simulink model "sldemo_foucault"  (Simulink 10.0)
settings: Solver=ode23t  StartTime=0.0  StopTime=3600  FixedStep=.1  RelTol=1e-5  EnableMultiTasking=on
PreLoadFcn:
  | sldemo_foucault_data;
undefined symbols (not defined in the file): g, initial_x, initial_xdot, initial_y, initial_ydot, L, lambda, Omega
CloseFcn:
  | close(findobj('Tag','CloseMe'));
settings Model: Creator=The MathWorks, Inc.  LastModifiedBy=bhisma
settings DataIOCC: SaveFormat=StructureWithTime  SaveOutput=off  SaveTime=off  ReturnWorkspaceOutputs=on  ReturnWorkspaceOutputsName=sldemo_foucault_output
settings OptimizationCC: ExpressionDepthLimit=2147483647  InitFltsAndDblsToZero=on
settings DebuggingCC: SaveWithParameterizedLinksMsg=none  SignalResolutionControl=TryResolveAllWithWarning  FcnCallInpInsideContextMsg=warning  AllowSymbolicDim=off  StateNameClashWarn=warning
settings SFSimCC: CustomCodeUndefinedFunction=FilterOut
settings GRTTargetCC: TargetFcnLib=ansi_tfl_tmw.mat  GeneratePreprocessorConditionals=Disable all
settings ConfigComp: CovExternalEMLEnable=off

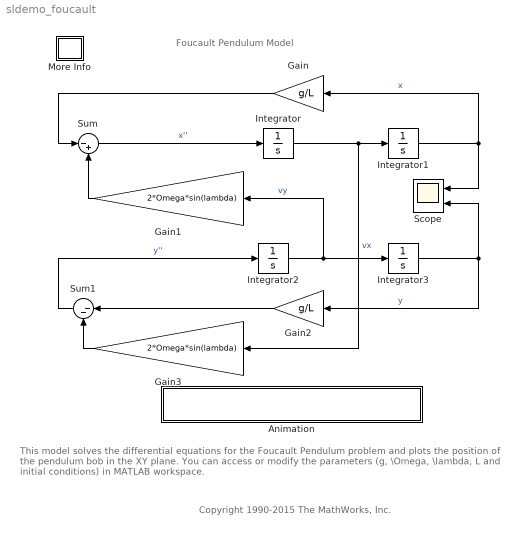
== system sldemo_foucault ==
  note: This model solves the differential equations for the Foucault Pendulum problem
      | and plots the position of the pendulum bob in the XY plane. You can access or modify
      | the parameters (g, \Omega, \lambda, L and initial conditions) in MATLAB workspace.
  note: Foucault Pendulum Model
  note: Copyright 1990-2015 The MathWorks, Inc.
  Animation : Subsystem
      settings: OpenFcn=|
      | if exist('sldemo_foucault_output','var')
      |    sldemo_foucault_animate;
      | else
      |    display('sldemo_foucault_output not found');
      |    display('Please run the simulation and then animate the results');
      | end
      mask Display: disp('Double Click Here to Animate Results')
  Gain : Gain  Gain=g/L
  Gain1 : Gain  Gain=2*Omega*sin(lambda)
  Gain2 : Gain  Gain=g/L
  Gain3 : Gain  Gain=2*Omega*sin(lambda)
  Integrator : Integrator  InitialCondition=initial_xdot
  Integrator1 : Integrator  InitialCondition=initial_x
  Integrator2 : Integrator  InitialCondition=initial_ydot
  Integrator3 : Integrator  InitialCondition=initial_y
  More Info : Subsystem
      settings: OpenFcn=showExample('simulink_general/sldemo_foucaultExample')
      mask Display: disp('?')
  Scope : Scope  NumInputPorts=2
  Sum : Sum  Inputs=|-+
  Sum1 : Sum  Inputs=|--
  wires:
  Integrator/1 -> Integrator1/1, Gain3/1  "vx"
  Integrator1/1 -> Scope/1, Gain/1  "x"
  Sum/1 -> Integrator/1  "x''"
  Gain/1 -> Sum/1
  Gain1/1 -> Sum/2
  Integrator2/1 -> Integrator3/1, Gain1/1  "vy"
  Gain2/1 -> Sum1/1
  Gain3/1 -> Sum1/2
  Sum1/1 -> Integrator2/1  "y''"
  Integrator3/1 -> Gain2/1, Scope/2  "y"

== system sldemo_foucault/Animation ==

== system sldemo_foucault/More Info ==
